simulink model "dbe_xaui_corr_32X"  (Simulink 7.1)
settings: Solver=ode45  StartTime=0.0  StopTime=1000  RelTol=1e-3
undefined symbols (not defined in the file or in its folder): iBOB
libraries: xbsIndex_r4 x455, xps_library x46, casper_library_misc x12, casper_library_sources x2, gavrt_library x1, simulink x1, casper_library_scopes x1
(part 1 of 4)
settings Model: Creator=rprimian  LastModifiedBy=Rurik A Primiani
settings DebuggingCC: SaveWithParameterizedLinksMsg=none  SignalResolutionControl=TryResolveAllWithWarning  MultiTaskDSMMsg=warning  MultiTaskCondExecSysMsg=none  StrictBusMsg=None
settings RTWCC: IncludeERTFirstTime=on
settings GRTTargetCC: TargetFcnLib=ansi_tfl_tmw.mat

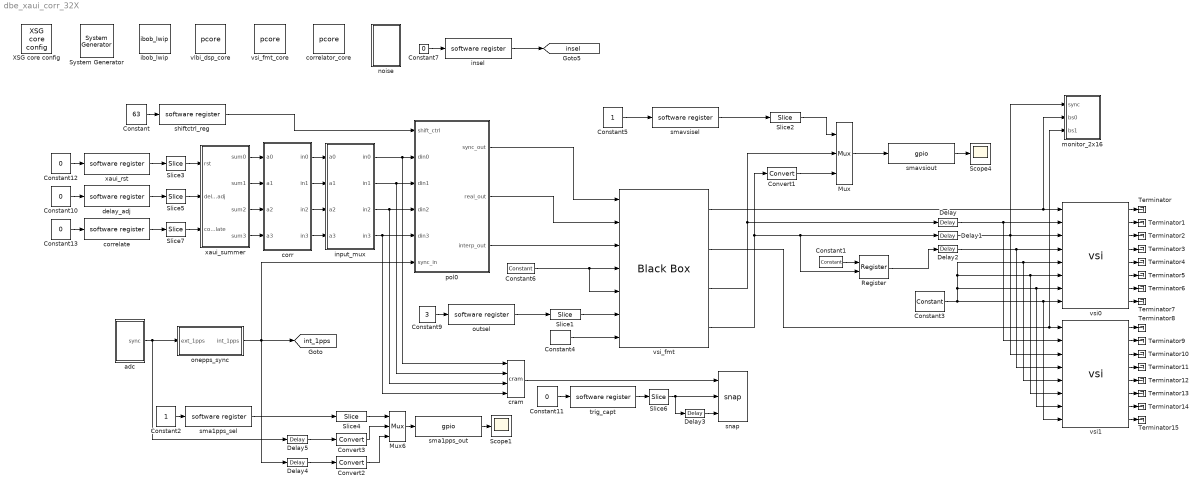
== system dbe_xaui_corr_32X ==
  " System Generator" : xbsIndex_r4/ System Generator  Tag=genX  SystemSampleTime=-1  xilinxfamily=virtex2p  part=xc2vp50  speed=-7  package=ff1152  synthesis_tool=XST  clock_wrapper=Clock Enables  directory=./dbe_xaui_corr_32X/sysgen  testbench=off  simulink_period=1  sysclk_period=3.9063  dcm_input_clock_period=10  incr_netlist=off  trim_vbits=Everywhere in SubSystem  dbl_ovrd=According to Block Masks  core_generation=According to Block Masks  run_coregen=off  deprecated_control=off  eval_field=0  block_type=sysgen
      settings: block_version=11.3
  Constant : Constant  Value=63  OutDataType=sfix(16)  OutScaling=2^0
  Constant1 : xbsIndex_r4/Constant  arith_type=Unsigned  const=1  n_bits=1  bin_pt=0  explicit_period=on  period=1  equ=P=C  opselect=C  inp2=PCIN>>17  opr=+  inp1=P  carry=CIN  dbl_ovrd=off  block_type=constant
      settings: block_version=11.3
  Constant{10..13} (4 alike) : Constant  Value=0  OutDataType=fixdt(1, 16)  OutScaling=2^0
  Constant2 : Constant  OutDataType=sfix(16)  OutScaling=2^0
  Constant3 : xbsIndex_r4/Constant  arith_type=Unsigned  const=0  n_bits=1  bin_pt=0  explicit_period=on  period=1  equ=P=C  opselect=C  inp2=PCIN>>17  opr=+  inp1=P  carry=CIN  dbl_ovrd=off  block_type=constant
      settings: block_version=11.3
  Constant4 : xbsIndex_r4/Constant  arith_type=Unsigned  const=6  n_bits=3  bin_pt=0  explicit_period=on  period=1  equ=P=C  opselect=C  inp2=PCIN>>17  opr=+  inp1=P  carry=CIN  dbl_ovrd=off  block_type=constant
      settings: block_version=11.3
  Constant5 : Constant  OutDataType=sfix(16)  OutScaling=2^0
  Constant6 : xbsIndex_r4/Constant  arith_type=Unsigned  const=0  n_bits=4  bin_pt=0  explicit_period=on  period=1  equ=P=C  opselect=C  inp2=PCIN>>17  opr=+  inp1=P  carry=CIN  dbl_ovrd=off  block_type=constant
      settings: block_version=11.3
  Constant7 : Constant  Value=0
  Constant9 : Constant  Value=3  OutDataType=sfix(16)  OutScaling=2^0
  Convert1 : xbsIndex_r4/Convert  arith_type=Unsigned  n_bits=1  bin_pt=0  quantization=Truncate  overflow=Wrap  latency=0  dbl_ovrd=off  pipeline=off  block_type=convert
      settings: xl_area=[0, 0, 0, 0, 0, 0, 0]  block_version=11.3
  Convert2 : xbsIndex_r4/Convert  arith_type=Unsigned  n_bits=1  bin_pt=0  quantization=Truncate  overflow=Wrap  latency=0  dbl_ovrd=off  pipeline=off  block_type=convert
      settings: xl_area=[0, 0, 0, 0, 0, 0, 0]  block_version=11.3
  Convert3 : xbsIndex_r4/Convert  arith_type=Unsigned  n_bits=1  bin_pt=0  quantization=Truncate  overflow=Wrap  latency=0  dbl_ovrd=off  pipeline=off  block_type=convert
      settings: xl_area=[0, 0, 0, 0, 0, 0, 0]  block_version=11.3
  Delay{,1,4..5} (4 alike) : xbsIndex_r4/Delay  en=off  latency=1  dbl_ovrd=off  reg_retiming=off  block_type=delay
      settings: xl_area=[0, 0, 0, 0, 0, 0, 0]  block_version=11.3
  Delay2 : xbsIndex_r4/Delay  en=off  latency=0  dbl_ovrd=off  reg_retiming=off  block_type=delay
      settings: xl_area=[0, 0, 0, 0, 0, 0, 0]  block_version=11.3
  Delay3 : xbsIndex_r4/Delay  en=off  latency=8  dbl_ovrd=off  reg_retiming=off  block_type=delay
      settings: xl_area=[0, 0, 0, 0, 0, 0, 0]  block_version=11.3
  Mux : xbsIndex_r4/Mux  inputs=2  en=off  latency=0  precision=Full  arith_type="Signed  (2's comp)"  n_bits=8  bin_pt=2  quantization=Truncate  overflow=Wrap  dbl_ovrd=off  block_type=mux
      settings: xl_area=[0, 0, 0, 0, 0, 0, 0]  block_version=11.3
  Mux6 : xbsIndex_r4/Mux  inputs=2  en=off  latency=0  precision=Full  arith_type="Signed  (2's comp)"  n_bits=8  bin_pt=2  quantization=Truncate  overflow=Wrap  dbl_ovrd=off  block_type=mux
      settings: xl_area=[0, 0, 0, 0, 0, 0, 0]  block_version=11.3
  Register : xbsIndex_r4/Register  init=0  rst=off  en=on  dbl_ovrd=off  block_type=register
      settings: xl_area=[0, 0, 0, 0, 0, 0, 0]  block_version=11.3
  Scope1 : Scope
      settings: TimeRange=94.87951807228916  YMin=0.5138408304498272  YMax=0.5276816608996542
  Scope4 : Scope
      settings: TimeRange=94.87951807228916  YMin=0.5138408304498272  YMax=0.5276816608996542  SaveName=ScopeData2
  Slice1 : xbsIndex_r4/Slice  nbits=2  boolean_output=off  mode=Lower Bit Location + Width  bit1=0  base1=MSB of Input  bit0=0  base0=LSB of Input  dbl_ovrd=off  block_type=slice
      settings: block_version=11.3
  Slice2 : xbsIndex_r4/Slice  nbits=1  boolean_output=off  mode=Lower Bit Location + Width  bit1=0  base1=MSB of Input  bit0=0  base0=LSB of Input  dbl_ovrd=off  block_type=slice
      settings: block_version=11.3
  Slice3 : xbsIndex_r4/Slice  nbits=1  boolean_output=on  mode=Lower Bit Location + Width  bit1=0  base1=MSB of Input  bit0=0  base0=LSB of Input  dbl_ovrd=off  block_type=slice
      settings: infoedit="Extracts a given range of bits from each input sample and presents it at the output.  The output type is ordinarily unsigned with binary point at zero, but can be Boolean when the slice is one bit wide.<P><P>Hardware notes: In hardware this block costs nothing."  block_version=10.1.3
  Slice4 : xbsIndex_r4/Slice  nbits=1  boolean_output=off  mode=Lower Bit Location + Width  bit1=0  base1=MSB of Input  bit0=0  base0=LSB of Input  dbl_ovrd=off  block_type=slice
      settings: block_version=11.3
  Slice5 : xbsIndex_r4/Slice  nbits=4  boolean_output=off  mode=Lower Bit Location + Width  bit1=0  base1=MSB of Input  bit0=0  base0=LSB of Input  dbl_ovrd=off  block_type=slice
      settings: infoedit="Extracts a given range of bits from each input sample and presents it at the output.  The output type is ordinarily unsigned with binary point at zero, but can be Boolean when the slice is one bit wide.<P><P>Hardware notes: In hardware this block costs nothing."  block_version=10.1.3
  Slice6 : xbsIndex_r4/Slice  nbits=4  boolean_output=on  mode=Lower Bit Location + Width  bit1=0  base1=MSB of Input  bit0=0  base0=LSB of Input  dbl_ovrd=off  block_type=slice
      settings: infoedit="Extracts a given range of bits from each input sample and presents it at the output.  The output type is ordinarily unsigned with binary point at zero, but can be Boolean when the slice is one bit wide.<P><P>Hardware notes: In hardware this block costs nothing."  block_version=10.1.3
  Slice7 : xbsIndex_r4/Slice  nbits=1  boolean_output=on  mode=Lower Bit Location + Width  bit1=0  base1=MSB of Input  bit0=0  base0=LSB of Input  dbl_ovrd=off  block_type=slice
      settings: infoedit="Extracts a given range of bits from each input sample and presents it at the output.  The output type is ordinarily unsigned with binary point at zero, but can be Boolean when the slice is one bit wide.<P><P>Hardware notes: In hardware this block costs nothing."  block_version=10.1.3
  Terminator{,1..15} (16 alike) : Terminator
  XSG core config : xps_library/XSG core config  Tag=xps:xsg  SystemSampleTime=-1  hw_sys=iBOB  ibob_linux=off  clk_src=adc0_clk  iBOB_clk_src=adc0_clk  BEE2_ctrl_clk_src=sys_clk  BEE2_usr_clk_src=sys_clk  ROACH_clk_src=adc0_clk  CORR_clk_src=sys_clk  gpio_clk_io_group=iBOB:gpio0  gpio_clk_bit_index=0  clk_rate=256  sample_period=1  synthesis_tool=XST  mpc_type=powerpc405
  adc : Subsystem
  corr : Subsystem
  correlate : xps_library/software register  Tag=xps:sw_reg  SystemSampleTime=-1  io_dir=From Processor  arith_type=Unsigned  bitwidth=32  bin_pt=0  sample_period=1  gw_name=dbe_xaui_corr_32X_correlate_user_data_out
      link override dbe_xaui_align_user_data_out: arith_type=Unsigned  n_bits=32  bin_pt=0  period=1
      link override dbe_xaui_corr_32X_correlate_user_data_out: arith_type=Unsigned  n_bits=32  bin_pt=0  period=1
      link override dbe_xaui_corr_correlate_user_data_out: arith_type=Unsigned  n_bits=32  bin_pt=0  period=1
      link override dbe_xaui_correlate_user_data_out: arith_type=Unsigned  n_bits=32  bin_pt=0  period=1
      link override dbe_xaui_realign_user_data_out: arith_type=Unsigned  n_bits=32  bin_pt=0  period=1
      link override xaui_rx_reset_user_data_out: arith_type=Unsigned  n_bits=32  bin_pt=0  period=1
  correlator_core : xps_library/pcore  Tag=xps:pcore  SystemSampleTime=-1  pcore_path=./correlator_core/correlator_core.ngc
  cram : gavrt_library/cram  SystemSampleTime=-1  num_slice=4
  delay_adj : xps_library/software register  Tag=xps:sw_reg  SystemSampleTime=-1  io_dir=From Processor  arith_type=Unsigned  bitwidth=32  bin_pt=0  sample_period=1  gw_name=dbe_xaui_corr_32X_delay_adj_user_data_out
      link override dbe_xaui_corr_32X_delay_adj_user_data_out: arith_type=Unsigned  n_bits=32  bin_pt=0  period=1
      link override dbe_xaui_corr_delay_adj_user_data_out: arith_type=Unsigned  n_bits=32  bin_pt=0  period=1
      link override dbe_xaui_delay_adj_user_data_out: arith_type=Unsigned  n_bits=32  bin_pt=0  period=1
      link override dbe_xaui_realign_user_data_out: arith_type=Unsigned  n_bits=32  bin_pt=0  period=1
      link override xaui_rx_reset_user_data_out: arith_type=Unsigned  n_bits=32  bin_pt=0  period=1
  ibob_lwip : xps_library/ibob_lwip  SystemSampleTime=-1
      link override macbits/convert: arith_type=Unsigned  n_bits=32  bin_pt=0
      link override machdr/dbe_xaui_corr_32X_ibob_lwip_machdr_gateway: arith_type=Unsigned  n_bits=20  bin_pt=0  period=sample_period
      link override machdr/dbe_xaui_corr_ibob_lwip_machdr_gateway: arith_type=Unsigned  n_bits=20  bin_pt=0  period=sample_period
  input_mux : Subsystem
  insel : xps_library/software register  Tag=xps:sw_reg  SystemSampleTime=-1  io_dir=From Processor  arith_type=Unsigned  bitwidth=32  bin_pt=0  sample_period=1  gw_name=dbe_xaui_corr_32X_insel_user_data_out
      link override dbe_adc_single_insel_user_data_out: arith_type=Unsigned  n_bits=32  bin_pt=0  period=1
      link override dbe_adc_single_shiftctrl_reg_user_data_out: arith_type=Unsigned  n_bits=32  bin_pt=0  period=1
      link override dbe_xaui_corr_32X_insel_user_data_out: arith_type=Unsigned  n_bits=32  bin_pt=0  period=1
      link override vlbipfb2_m3_ibob_shiftctrl_reg_user_data_out: arith_type=Unsigned  n_bits=32  bin_pt=0  period=1
      link override vlbipfb2_m3_roach_shiftctrl_reg_user_data_out: arith_type=Unsigned  n_bits=32  bin_pt=0  period=1
  monitor_2x16 : Subsystem  mask{sample_width=2}
      mask prompts: sample_width "Sample width"
  noise : Subsystem
  onepps_sync : Subsystem
  outsel : xps_library/software register  Tag=xps:sw_reg  SystemSampleTime=-1  io_dir=From Processor  arith_type=Unsigned  bitwidth=32  bin_pt=0  sample_period=1  gw_name=dbe_xaui_corr_32X_outsel_user_data_out
      link override dbe_adc_single_output_sel_user_data_out: arith_type=Unsigned  n_bits=32  bin_pt=0  period=1
      link override dbe_xaui_corr_32X_outsel_user_data_out: arith_type=Unsigned  n_bits=32  bin_pt=0  period=1
      link override vlbipfb2_m3_ibob_output_sel_user_data_out: arith_type=Unsigned  n_bits=32  bin_pt=0  period=1
      link override vlbipfb2_m3_roach_output_sel_user_data_out: arith_type=Unsigned  n_bits=32  bin_pt=0  period=1
  pol0 : Subsystem
  shiftctrl_reg : xps_library/software register  Tag=xps:sw_reg  SystemSampleTime=-1  io_dir=From Processor  arith_type=Unsigned  bitwidth=32  bin_pt=0  sample_period=1  gw_name=dbe_xaui_corr_32X_shiftctrl_reg_user_data_out
      link override dbe_xaui_corr_32X_shiftctrl_reg_user_data_out: arith_type=Unsigned  n_bits=32  bin_pt=0  period=1
      link override dbe_xaui_corr_shiftctrl_reg_user_data_out: arith_type=Unsigned  n_bits=32  bin_pt=0  period=1
      link override dbe_xaui_shiftctrl_reg_user_data_out: arith_type=Unsigned  n_bits=32  bin_pt=0  period=1
      link override vlbipfb2_m3_ibob_shiftctrl_reg_user_data_out: arith_type=Unsigned  n_bits=32  bin_pt=0  period=1
      link override vlbipfb2_m3_roach_shiftctrl_reg_user_data_out: arith_type=Unsigned  n_bits=32  bin_pt=0  period=1
  sma1pps_out : xps_library/gpio  Tag=xps:gpio  SystemSampleTime=-1  io_group=iBOB:sma  io_dir=out  arith_type=Unsigned  bitwidth=1  bin_pt=0  bit_index=0  sample_period=1  use_single_ended=off  use_ddr=off  reg_iob=on  reg_clk_phase=0  termination=None
      link override convert: arith_type=Unsigned  n_bits=1  bin_pt=0
  sma1pps_sel : xps_library/software register  Tag=xps:sw_reg  SystemSampleTime=-1  io_dir=From Processor  arith_type=Unsigned  bitwidth=32  bin_pt=0  sample_period=1  gw_name=dbe_xaui_corr_32X_sma1pps_sel_user_data_out
      link override dbe_xaui_corr_32X_sma1pps_sel_user_data_out: arith_type=Unsigned  n_bits=32  bin_pt=0  period=1
      link override dbe_xaui_corr_sma1pps_sel_user_data_out: arith_type=Unsigned  n_bits=32  bin_pt=0  period=1
      link override dbe_xaui_corr_smasel_user_data_out: arith_type=Unsigned  n_bits=32  bin_pt=0  period=1
      link override dbe_xaui_smasel_user_data_out: arith_type=Unsigned  n_bits=32  bin_pt=0  period=1
      link override vlbipfb2_m3_ibob_smasel_user_data_out: arith_type=Unsigned  n_bits=32  bin_pt=0  period=1
      link override vlbipfb2_m3_roach_smasel_user_data_out: arith_type=Unsigned  n_bits=32  bin_pt=0  period=1
  smavsiout : xps_library/gpio  Tag=xps:gpio  SystemSampleTime=-1  io_group=iBOB:sma  io_dir=out  arith_type=Unsigned  bitwidth=1  bin_pt=0  bit_index=1  sample_period=1  use_single_ended=off  use_ddr=off  reg_iob=on  reg_clk_phase=0  termination=None
      link override convert: arith_type=Unsigned  n_bits=1  bin_pt=0
  smavsisel : xps_library/software register  Tag=xps:sw_reg  SystemSampleTime=-1  io_dir=From Processor  arith_type=Unsigned  bitwidth=32  bin_pt=0  sample_period=1  gw_name=dbe_xaui_corr_32X_smavsisel_user_data_out
      link override dbe_adc_single_smasel_user_data_out: arith_type=Unsigned  n_bits=32  bin_pt=0  period=1
      link override dbe_xaui_corr_32X_smavsisel_user_data_out: arith_type=Unsigned  n_bits=32  bin_pt=0  period=1
      link override vlbipfb2_m3_ibob_smasel_user_data_out: arith_type=Unsigned  n_bits=32  bin_pt=0  period=1
      link override vlbipfb2_m3_roach_smasel_user_data_out: arith_type=Unsigned  n_bits=32  bin_pt=0  period=1
  snap : casper_library_scopes/snap  SystemSampleTime=-1  nsamples=11
      link override addr/convert: arith_type=Unsigned  n_bits=32  bin_pt=0
      link override bram/convert_din: arith_type=Unsigned
      link override bram/dbe_xaui_corr_32X_snap_bram_data_out: arith_type=Unsigned
      link override bram/dbe_xaui_corr_snap_bram_data_out: arith_type=Unsigned
      link override bram/dbe_xaui_snap_bram_data_out: arith_type=Unsigned
      link override bram/mem/sim_data_in: arith_type=Unsigned
      link override ctrl/dbe_xaui_corr_32X_snap_ctrl_user_data_out: arith_type=Unsigned  n_bits=32  bin_pt=0  period=1
      link override ctrl/dbe_xaui_corr_snap_ctrl_user_data_out: arith_type=Unsigned  n_bits=32  bin_pt=0  period=1
      link override ctrl/dbe_xaui_snap_ctrl_user_data_out: arith_type=Unsigned  n_bits=32  bin_pt=0  period=1
  trig_capt : xps_library/software register  Tag=xps:sw_reg  SystemSampleTime=-1  io_dir=From Processor  arith_type=Unsigned  bitwidth=32  bin_pt=0  sample_period=1  gw_name=dbe_xaui_corr_32X_trig_capt_user_data_out
      link override dbe_xaui_corr_32X_trig_capt_user_data_out: arith_type=Unsigned  n_bits=32  bin_pt=0  period=1
      link override dbe_xaui_corr_trig_capt_user_data_out: arith_type=Unsigned  n_bits=32  bin_pt=0  period=1
      link override dbe_xaui_delay_adj_user_data_out: arith_type=Unsigned  n_bits=32  bin_pt=0  period=1
      link override dbe_xaui_realign_user_data_out: arith_type=Unsigned  n_bits=32  bin_pt=0  period=1
      link override dbe_xaui_trig_capt_user_data_out: arith_type=Unsigned  n_bits=32  bin_pt=0  period=1
      link override xaui_rx_reset_user_data_out: arith_type=Unsigned  n_bits=32  bin_pt=0  period=1
  vlbi_dsp_core : xps_library/pcore  Tag=xps:pcore  SystemSampleTime=-1  pcore_path=vlbi_dsp_core/vlbi_dsp_core.ngc
  vsi0 : xps_library/vsi  Tag=xps:vsi  SystemSampleTime=-1  connector=MDR  arith_type=Unsigned  bin_pt=0  sample_period=1
      link override convert_bs: arith_type=Unsigned  n_bits=32  bin_pt=0
  vsi1 : xps_library/vsi  Tag=xps:vsi  SystemSampleTime=-1  connector=ZDOK 1  arith_type=Unsigned  bin_pt=0  sample_period=1
      link override convert_bs: arith_type=Unsigned  n_bits=32  bin_pt=0
  vsi_fmt : xbsIndex_r4/Black Box  init_code=vsi_fmt_core_config  sim_method=Inactive  block_type=blackbox2
      settings: infoedit="Incorporates black box HDL and simulation model into a System Generator design.<P><P>You must supply a Black Box with certain information about the HDL component you would like to bring into System Generator. This information is provided through a Matlab function.<P><P>When \"Simulation mode\" is set to \"Inactive\", you will typically want to provide a separate simulation model by using a Simulation Multiplexer.<P>When \"Simulation mode\" is set to \"External co-simulator\", you must include a ModelSim block in the design."  block_version=10.1.3
  vsi_fmt_core : xps_library/pcore  Tag=xps:pcore  SystemSampleTime=-1  pcore_path=vsi_fmt_core/vsi_fmt_core.ngc
  xaui_rst : xps_library/software register  Tag=xps:sw_reg  SystemSampleTime=-1  io_dir=From Processor  arith_type=Unsigned  bitwidth=32  bin_pt=0  sample_period=1  gw_name=dbe_xaui_corr_32X_xaui_rst_user_data_out
      link override dbe_xaui_corr_32X_xaui_rst_user_data_out: arith_type=Unsigned  n_bits=32  bin_pt=0  period=1
      link override dbe_xaui_corr_xaui_rst_user_data_out: arith_type=Unsigned  n_bits=32  bin_pt=0  period=1
      link override dbe_xaui_xaui_rst_user_data_out: arith_type=Unsigned  n_bits=32  bin_pt=0  period=1
      link override xaui_rx_reset_user_data_out: arith_type=Unsigned  n_bits=32  bin_pt=0  period=1
  xaui_summer : Subsystem
  tag scope: insel=global, int_1pps=global
  wires:
  Constant/1 -> shiftctrl_reg/1
  adc/1(sync) -> onepps_sync/1(ext_1pps), Delay5/1
  shiftctrl_reg/1 -> pol0/1(shift_ctrl)
  onepps_sync/1(int_1pps) -> pol0/6(sync_in), [int_1pps], Delay4/1
  Constant12/1 -> xaui_rst/1
  xaui_rst/1 -> Slice3/1
  Slice3/1 -> xaui_summer/1(rst)
  Constant10/1 -> delay_adj/1
  delay_adj/1 -> Slice5/1
  Slice5/1 -> xaui_summer/2(delay_adj)
  Constant13/1 -> correlate/1
  correlate/1 -> Slice7/1
  Slice7/1 -> xaui_summer/3(correlate)
  Mux6/1 -> sma1pps_out/1
  sma1pps_sel/1 -> Slice4/1
  Constant2/1 -> sma1pps_sel/1
  Convert2/1 -> Mux6/3
  Slice4/1 -> Mux6/1
  sma1pps_out/1 -> Scope1/1
  Convert3/1 -> Mux6/2
  vsi_fmt/4 -> Delay1/1, Register/2, Convert1/1
  Constant3/1 -> vsi0/6, vsi1/6, vsi0/5, vsi1/5, vsi0/7, vsi1/7, vsi0/8, vsi1/8
  Constant1/1 -> Register/1
  Register/1 -> Delay2/1
  Mux/1 -> smavsiout/1
  smavsisel/1 -> Slice2/1
  Constant5/1 -> smavsisel/1
  Convert1/1 -> Mux/3
  Slice2/1 -> Mux/1
  smavsiout/1 -> Scope4/1
  Constant9/1 -> outsel/1
  Delay/1 -> vsi0/2, vsi1/2
  Delay1/1 -> monitor_2x16/1(sync), vsi0/3, vsi1/3
  Delay2/1 -> vsi0/4, vsi1/4
  input_mux/1(in0) -> pol0/2(din0), cram/1
  input_mux/2(in1) -> pol0/3(din1), cram/2
  input_mux/3(in2) -> pol0/4(din2), cram/3
  input_mux/4(in3) -> pol0/5(din3), cram/4
  vsi_fmt/3 -> Mux/2, Delay/1
  vsi_fmt/1 -> vsi0/1, monitor_2x16/2(bs0)
  vsi_fmt/2 -> monitor_2x16/3(bs1), vsi1/1
  pol0/1(sync_out) -> vsi_fmt/1
  pol0/2(real_out) -> vsi_fmt/2
  pol0/3(interp_out) -> vsi_fmt/3
  Constant6/1 -> vsi_fmt/4, vsi_fmt/5
  outsel/1 -> Slice1/1
  Constant4/1 -> vsi_fmt/7
  Slice1/1 -> vsi_fmt/6
  cram/1 -> snap/1
  Constant11/1 -> trig_capt/1
  trig_capt/1 -> Slice6/1
  Delay3/1 -> snap/3
  Slice6/1 -> snap/2, Delay3/1
  Constant7/1 -> insel/1
  insel/1 -> [insel]
  vsi0/1 -> Terminator/1
  vsi0/2 -> Terminator1/1
  vsi0/3 -> Terminator2/1
  vsi0/4 -> Terminator3/1
  vsi0/5 -> Terminator4/1
  vsi0/6 -> Terminator5/1
  vsi0/7 -> Terminator6/1
  vsi0/8 -> Terminator7/1
  vsi1/1 -> Terminator8/1
  vsi1/2 -> Terminator9/1
  vsi1/3 -> Terminator10/1
  vsi1/4 -> Terminator11/1
  vsi1/5 -> Terminator12/1
  vsi1/6 -> Terminator13/1
  vsi1/7 -> Terminator14/1
  vsi1/8 -> Terminator15/1
  Delay5/1 -> Convert3/1
  Delay4/1 -> Convert2/1
  xaui_summer/1(sum0) -> corr/1(a0)
  xaui_summer/2(sum1) -> corr/2(a1)
  xaui_summer/3(sum2) -> corr/3(a2)
  xaui_summer/4(sum3) -> corr/4(a3)
  corr/1(in0) -> input_mux/1(a0)
  corr/2(in1) -> input_mux/2(a1)
  corr/3(in2) -> input_mux/3(a2)
  corr/4(in3) -> input_mux/4(a3)

== system dbe_xaui_corr_32X/adc ==
  Constant10 : Constant  OutDataType=sfix(16)  OutScaling=2^0  SampleTime=0.25
  Pulse Generator : DiscretePulseGenerator  Period=2560  PhaseDelay=20  SampleTime=0.25
  Sine Wave : Sin  Amplitude=.8  Frequency=2*pi*119/256  Samples=2*pi*129/1024  SampleTime=1/4
  Sine Wave1 : Sin  Amplitude=.8  Frequency=2*pi*77/256  Samples=2*pi*129/1024  SampleTime=1/4
  Terminator{,1..6,8..12} (12 alike) : Terminator
  adc : xps_library/adc  Tag=xps:adc  SystemSampleTime=-1  adc_brd=adc0  adc_clk_rate=1024  adc_interleave=off  sample_period=1
  sync : Outport
  tag scope: adc0=global, adc1=global, adc2=global, adc3=global
  wires:
  Constant10/1 -> adc/4
  Pulse Generator/1 -> adc/3
  Sine Wave/1 -> adc/1
  adc/9 -> Terminator/1
  adc/10 -> Terminator1/1
  adc/11 -> Terminator3/1
  adc/12 -> Terminator8/1
  adc/14 -> Terminator9/1
  adc/15 -> Terminator10/1
  adc/16 -> Terminator11/1
  adc/17 -> Terminator12/1
  Sine Wave1/1 -> adc/2
  adc/5 -> Terminator2/1
  adc/6 -> Terminator4/1
  adc/7 -> Terminator5/1
  adc/8 -> Terminator6/1
  adc/1 -> [adc0]
  adc/2 -> [adc1]
  adc/3 -> [adc2]
  adc/4 -> [adc3]
  adc/13 -> sync/1

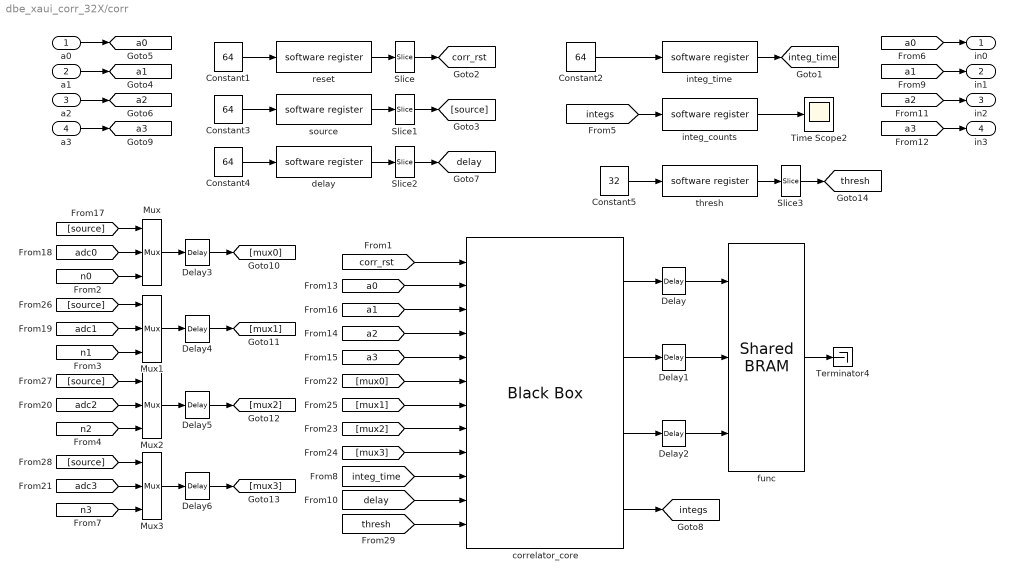
== system dbe_xaui_corr_32X/corr ==
  a0 : Inport
  a1 : Inport  Port=2
  a2 : Inport  Port=3
  a3 : Inport  Port=4
  Constant{1..4} (4 alike) : Constant  Value=64  OutDataType=fixdt(1, 16)  OutScaling=2^0
  Constant5 : Constant  Value=32  OutDataType=fixdt(1, 16)  OutScaling=2^0
  Delay{,1..6} (7 alike) : xbsIndex_r4/Delay  en=off  latency=1  dbl_ovrd=off  reg_retiming=off  block_type=delay
  Mux{,1..3} (4 alike) : xbsIndex_r4/Mux  inputs=2  en=off  latency=1  precision=Full  arith_type=Unsigned  n_bits=16  bin_pt=14  quantization=Truncate  overflow=Wrap  dbl_ovrd=off  block_type=mux
  Slice : xbsIndex_r4/Slice  nbits=1  boolean_output=on  mode=Lower Bit Location + Width  bit1=0  base1=MSB of Input  bit0=0  base0=LSB of Input  dbl_ovrd=off  block_type=slice
      settings: infoedit="Extracts a given range of bits from each input sample and presents it at the output.  The output type is ordinarily unsigned with binary point at zero, but can be Boolean when the slice is one bit wide.<P><P>Hardware notes: In hardware this block costs nothing."  block_version=10.1.3
  Slice1 : xbsIndex_r4/Slice  nbits=1  boolean_output=on  mode=Lower Bit Location + Width  bit1=0  base1=MSB of Input  bit0=0  base0=LSB of Input  dbl_ovrd=off  block_type=slice
      settings: infoedit="Extracts a given range of bits from each input sample and presents it at the output.  The output type is ordinarily unsigned with binary point at zero, but can be Boolean when the slice is one bit wide.<P><P>Hardware notes: In hardware this block costs nothing."  block_version=10.1.3
  Slice2 : xbsIndex_r4/Slice  nbits=11  boolean_output=off  mode=Lower Bit Location + Width  bit1=0  base1=MSB of Input  bit0=0  base0=LSB of Input  dbl_ovrd=off  block_type=slice
      settings: infoedit="Extracts a given range of bits from each input sample and presents it at the output.  The output type is ordinarily unsigned with binary point at zero, but can be Boolean when the slice is one bit wide.<P><P>Hardware notes: In hardware this block costs nothing."  block_version=10.1.3
  Slice3 : xbsIndex_r4/Slice  nbits=7  boolean_output=off  mode=Lower Bit Location + Width  bit1=0  base1=MSB of Input  bit0=0  base0=LSB of Input  dbl_ovrd=off  block_type=slice
      settings: infoedit="Extracts a given range of bits from each input sample and presents it at the output.  The output type is ordinarily unsigned with binary point at zero, but can be Boolean when the slice is one bit wide.<P><P>Hardware notes: In hardware this block costs nothing."  block_version=10.1.3
  Terminator4 : Terminator
  Time Scope2 : Scope
      settings: YMin=0  YMax=32.5  SaveName=ScopeData3  DataFormat=Structure
  correlator_core : xbsIndex_r4/Black Box  init_code=correlator_core_config  sim_method=Inactive  block_type=blackbox2
      settings: infoedit="Incorporates black box HDL and simulation model into a System Generator design.<P><P>You must supply a Black Box with certain information about the HDL component you would like to bring into System Generator. This information is provided through a Matlab function.<P><P>When \"Simulation mode\" is set to \"Inactive\", you will typically want to provide a separate simulation model by using a Simulation Multiplexer.<P>When \"Simulation mode\" is set to \"External co-simulator\", you must include a ModelSim block in the design."  block_version=10.1.3
  delay : xps_library/software register  Tag=xps:sw_reg  SystemSampleTime=-1  io_dir=From Processor  arith_type=Unsigned  bitwidth=32  bin_pt=0  sample_period=1  gw_name=dbe_xaui_corr_32X_corr_delay_user_data_out
      link override correlator_2bit_bee2_integ_time_user_data_out: arith_type=Unsigned  n_bits=32  bin_pt=0  period=1
      link override correlator_2bit_bee2_x2_integ_time_user_data_out: arith_type=Unsigned  n_bits=32  bin_pt=0  period=1
      link override correlator_2bit_ibob_integ_time_user_data_out: arith_type=Unsigned  n_bits=32  bin_pt=0  period=1
      link override dbe_xaui_corr_32X_corr_delay_user_data_out: arith_type=Unsigned  n_bits=32  bin_pt=0  period=1
      link override dbe_xaui_corr_corr_delay_user_data_out: arith_type=Unsigned  n_bits=32  bin_pt=0  period=1
      link override dbe_xaui_corr_corr_integ_time_user_data_out: arith_type=Unsigned  n_bits=32  bin_pt=0  period=1
      link override dbe_xaui_corr_corr_integ_user_data_out: arith_type=Unsigned  n_bits=32  bin_pt=0  period=1
      link override dbe_xaui_corr_new_corr_integ_user_data_out: arith_type=Unsigned  n_bits=32  bin_pt=0  period=1
  func : xps_library/Shared BRAM  Tag=xps:bram  SystemSampleTime=-1  arith_type="Signed  (2's comp)"  addr_width=11  data_width=32  data_bin_pt=0  init_vals=0  sample_rate=1
      link override convert_din: arith_type="Signed  (2's comp)"
      link override correlator_2bit_bee2_output_corr0_data_out: arith_type=Unsigned
      link override correlator_2bit_bee2_x2_output_corr01_data_out: arith_type=Unsigned
      link override correlator_2bit_bee2_x2_output_corr0_data_out: arith_type=Unsigned
      link override correlator_2bit_ibob_output_corr0_data_out: arith_type=Unsigned
      link override cross_correlator_test_corr_out_data_out: arith_type="Signed  (2's comp)"
      link override cross_correlator_test_input_data1_data_out: arith_type=Unsigned
      link override dbe_xaui_corr_32X_corr_func_data_out: arith_type="Signed  (2's comp)"
      link override dbe_xaui_corr_corr_func_data_out: arith_type="Signed  (2's comp)"
      link override dbe_xaui_corr_new_xaui_summer_summer_output_corr_data_out: arith_type="Signed  (2's comp)"
      link override dbe_xaui_corr_xaui_summer_summer_output_corr_data_out: arith_type="Signed  (2's comp)"
      link override mem/sim_data_in: arith_type="Signed  (2's comp)"
  integ_counts : xps_library/software register  Tag=xps:sw_reg  SystemSampleTime=-1  io_dir=To Processor  arith_type=Unsigned  bitwidth=32  bin_pt=0  sample_period=1  gw_name=dbe_xaui_corr_32X_corr_integ_counts_user_data_in
      link override convert: arith_type=Unsigned  n_bits=32  bin_pt=0
  integ_time : xps_library/software register  Tag=xps:sw_reg  SystemSampleTime=-1  io_dir=From Processor  arith_type=Unsigned  bitwidth=32  bin_pt=0  sample_period=1  gw_name=dbe_xaui_corr_32X_corr_integ_time_user_data_out
      link override correlator_2bit_bee2_integ_time_user_data_out: arith_type=Unsigned  n_bits=32  bin_pt=0  period=1
      link override correlator_2bit_bee2_x2_integ_time_user_data_out: arith_type=Unsigned  n_bits=32  bin_pt=0  period=1
      link override correlator_2bit_ibob_integ_time_user_data_out: arith_type=Unsigned  n_bits=32  bin_pt=0  period=1
      link override dbe_xaui_corr_32X_corr_integ_time_user_data_out: arith_type=Unsigned  n_bits=32  bin_pt=0  period=1
      link override dbe_xaui_corr_corr_integ_time_user_data_out: arith_type=Unsigned  n_bits=32  bin_pt=0  period=1
      link override dbe_xaui_corr_corr_integ_user_data_out: arith_type=Unsigned  n_bits=32  bin_pt=0  period=1
      link override dbe_xaui_corr_new_corr_integ_user_data_out: arith_type=Unsigned  n_bits=32  bin_pt=0  period=1
  reset : xps_library/software register  Tag=xps:sw_reg  SystemSampleTime=-1  io_dir=From Processor  arith_type=Unsigned  bitwidth=32  bin_pt=0  sample_period=1  gw_name=dbe_xaui_corr_32X_corr_reset_user_data_out
      link override correlator_2bit_bee2_integ_time_user_data_out: arith_type=Unsigned  n_bits=32  bin_pt=0  period=1
      link override correlator_2bit_bee2_x2_integ_time_user_data_out: arith_type=Unsigned  n_bits=32  bin_pt=0  period=1
      link override correlator_2bit_ibob_integ_time_user_data_out: arith_type=Unsigned  n_bits=32  bin_pt=0  period=1
      link override dbe_xaui_corr_32X_corr_reset_user_data_out: arith_type=Unsigned  n_bits=32  bin_pt=0  period=1
      link override dbe_xaui_corr_corr_integ_user_data_out: arith_type=Unsigned  n_bits=32  bin_pt=0  period=1
      link override dbe_xaui_corr_corr_reset_user_data_out: arith_type=Unsigned  n_bits=32  bin_pt=0  period=1
      link override dbe_xaui_corr_new_corr_integ_user_data_out: arith_type=Unsigned  n_bits=32  bin_pt=0  period=1
  source : xps_library/software register  Tag=xps:sw_reg  SystemSampleTime=-1  io_dir=From Processor  arith_type=Unsigned  bitwidth=32  bin_pt=0  sample_period=1  gw_name=dbe_xaui_corr_32X_corr_source_user_data_out
      link override correlator_2bit_bee2_integ_time_user_data_out: arith_type=Unsigned  n_bits=32  bin_pt=0  period=1
      link override correlator_2bit_bee2_x2_integ_time_user_data_out: arith_type=Unsigned  n_bits=32  bin_pt=0  period=1
      link override correlator_2bit_ibob_integ_time_user_data_out: arith_type=Unsigned  n_bits=32  bin_pt=0  period=1
      link override dbe_xaui_corr_32X_corr_source_user_data_out: arith_type=Unsigned  n_bits=32  bin_pt=0  period=1
      link override dbe_xaui_corr_corr_integ_time_user_data_out: arith_type=Unsigned  n_bits=32  bin_pt=0  period=1
      link override dbe_xaui_corr_corr_integ_user_data_out: arith_type=Unsigned  n_bits=32  bin_pt=0  period=1
      link override dbe_xaui_corr_corr_source_user_data_out: arith_type=Unsigned  n_bits=32  bin_pt=0  period=1
      link override dbe_xaui_corr_new_corr_integ_user_data_out: arith_type=Unsigned  n_bits=32  bin_pt=0  period=1
  thresh : xps_library/software register  Tag=xps:sw_reg  SystemSampleTime=-1  io_dir=From Processor  arith_type=Unsigned  bitwidth=32  bin_pt=0  sample_period=1  gw_name=dbe_xaui_corr_32X_corr_thresh_user_data_out
      link override correlator_2bit_bee2_integ_time_user_data_out: arith_type=Unsigned  n_bits=32  bin_pt=0  period=1
      link override correlator_2bit_bee2_x2_integ_time_user_data_out: arith_type=Unsigned  n_bits=32  bin_pt=0  period=1
      link override correlator_2bit_ibob_integ_time_user_data_out: arith_type=Unsigned  n_bits=32  bin_pt=0  period=1
      link override dbe_xaui_corr_32X_corr_thresh_user_data_out: arith_type=Unsigned  n_bits=32  bin_pt=0  period=1
      link override dbe_xaui_corr_corr_delay_user_data_out: arith_type=Unsigned  n_bits=32  bin_pt=0  period=1
      link override dbe_xaui_corr_corr_integ_time_user_data_out: arith_type=Unsigned  n_bits=32  bin_pt=0  period=1
      link override dbe_xaui_corr_corr_integ_user_data_out: arith_type=Unsigned  n_bits=32  bin_pt=0  period=1
      link override dbe_xaui_corr_corr_thresh_user_data_out: arith_type=Unsigned  n_bits=32  bin_pt=0  period=1
      link override dbe_xaui_corr_new_corr_integ_user_data_out: arith_type=Unsigned  n_bits=32  bin_pt=0  period=1
  in0 : Outport
  in1 : Outport  Port=2
  in2 : Outport  Port=3
  in3 : Outport  Port=4
  tag scope: a0=global, a1=global, a2=global, a3=global, corr_rst=global, delay=global, integ_time=global, integs=global, thresh=global
  wires:
  Constant2/1 -> integ_time/1
  integ_counts/1 -> Time Scope2/1
  integ_time/1 -> [integ_time]
  [integs] -> integ_counts/1
  func/1 -> Terminator4/1
  Constant1/1 -> reset/1
  reset/1 -> Slice/1
  Slice/1 -> [corr_rst]
  Constant3/1 -> source/1
  source/1 -> Slice1/1
  [corr_rst] -> correlator_core/1
  a0/1 -> [a0]
  a1/1 -> [a1]
  a2/1 -> [a2]
  a3/1 -> [a3]
  [a0] -> in0/1
  [a1] -> in1/1
  [a2] -> in2/1
  [a3] -> in3/1
  [a0] -> correlator_core/2
  [a1] -> correlator_core/3
  [a2] -> correlator_core/4
  [a3] -> correlator_core/5
  [n0] -> Mux/3
  [n1] -> Mux1/3
  [n2] -> Mux2/3
  [n3] -> Mux3/3
  [adc0] -> Mux/2
  [adc1] -> Mux1/2
  [adc2] -> Mux2/2
  [adc3] -> Mux3/2
  Mux/1 -> Delay3/1
  Mux1/1 -> Delay4/1
  Mux2/1 -> Delay5/1
  Mux3/1 -> Delay6/1
  [mux0] -> correlator_core/6
  [mux1] -> correlator_core/7
  [mux2] -> correlator_core/8
  [mux3] -> correlator_core/9
  [source] -> Mux/1
  [source] -> Mux1/1
  [source] -> Mux2/1
  Slice1/1 -> [source]
  [source] -> Mux3/1
  Constant4/1 -> delay/1
  delay/1 -> Slice2/1
  Slice2/1 -> [delay]
  correlator_core/1 -> Delay/1
  correlator_core/2 -> Delay1/1
  correlator_core/3 -> Delay2/1
  [integ_time] -> correlator_core/10
  [delay] -> correlator_core/11
  correlator_core/4 -> [integs]
  Delay/1 -> func/1
  Delay1/1 -> func/2
  Delay2/1 -> func/3
  [thresh] -> correlator_core/12
  Constant5/1 -> thresh/1
  thresh/1 -> Slice3/1
  Slice3/1 -> [thresh]
  Delay3/1 -> [mux0]
  Delay4/1 -> [mux1]
  Delay5/1 -> [mux2]
  Delay6/1 -> [mux3]

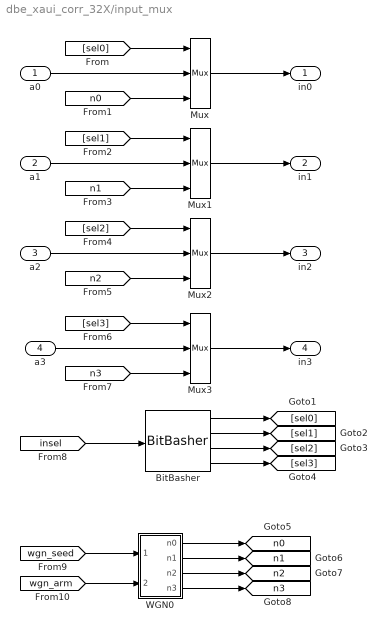
== system dbe_xaui_corr_32X/input_mux ==
  a0 : Inport
  a1 : Inport  Port=2
  a2 : Inport  Port=3
  a3 : Inport  Port=4
  BitBasher : xbsIndex_r4/BitBasher  bitexpr=|  display_expr=off  sr_1=1  arith_type1=Unsigned  bin_pt1=0  sr_2=2  arith_type2=Unsigned  bin_pt2=0  sr_3=3  arith_type3=Unsigned  bin_pt3=0  sr_4=4  arith_type4=Unsigned  bin_pt4=0  dbl_ovrd=off  block_type=bitbasher
      | <html><head><meta name="qrichtext" content="1" /><style type="text/css">
      | p, li { white-space: pre-wrap; }
      | </style></head><body style=" font-family:'MS Shell Dlg 2'; font-size:8.25pt; font-weight:400; font-style:normal;">
      | <p style=" margin-top:12px; margin-bottom:12px; margin-left:0px; margin-right:0px; -qt-block-indent:0; text-indent:0px; font-family:'MS Shell Dlg'; font-size:8pt;">sel0={insel[0]}<br />sel1={insel[1]}<br />sel2={insel[2]}<br />sel3={insel[3]}<br /></p></body></html>
      settings: block_version=10.1.3
  Mux{,1..3} (4 alike) : xbsIndex_r4/Mux  inputs=2  en=off  latency=0  precision=Full  arith_type=Unsigned  n_bits=16  bin_pt=14  quantization=Truncate  overflow=Wrap  dbl_ovrd=off  block_type=mux
  WGN0 : Subsystem
  in0 : Outport
  in1 : Outport  Port=2
  in2 : Outport  Port=3
  in3 : Outport  Port=4
  tag scope: n0=global, n1=global, n2=global, n3=global
  wires:
  Mux/1 -> in0/1
  BitBasher/1 -> [sel0]
  BitBasher/2 -> [sel1]
  BitBasher/3 -> [sel2]
  BitBasher/4 -> [sel3]
  [sel0] -> Mux/1
  WGN0/1(n0) -> [n0]
  WGN0/2(n1) -> [n1]
  WGN0/3(n2) -> [n2]
  WGN0/4(n3) -> [n3]
  a0/1 -> Mux/2
  [n0] -> Mux/3
  Mux1/1 -> in1/1
  [sel1] -> Mux1/1
  a1/1 -> Mux1/2
  [n1] -> Mux1/3
  Mux2/1 -> in2/1
  [sel2] -> Mux2/1
  a2/1 -> Mux2/2
  [n2] -> Mux2/3
  Mux3/1 -> in3/1
  [sel3] -> Mux3/1
  a3/1 -> Mux3/2
  [n3] -> Mux3/3
  [insel] -> BitBasher/1
  [wgn_seed] -> WGN0/1(seed)
  [wgn_arm] -> WGN0/2(arm)

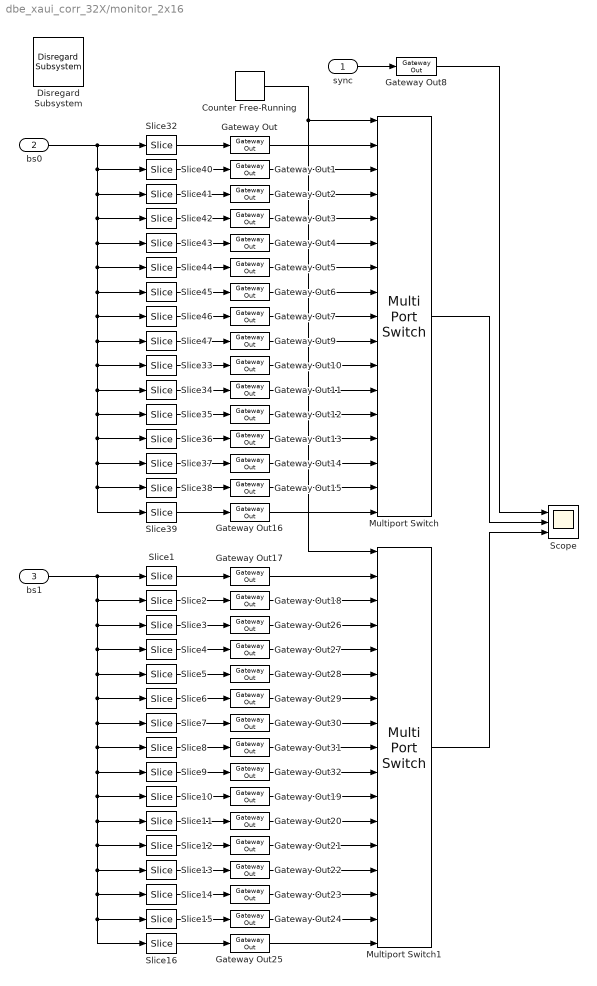
== system dbe_xaui_corr_32X/monitor_2x16 ==
  sync : Inport  OutDataType=sfix(16)  OutScaling=2^0
  bs0 : Inport  Port=2  OutDataType=sfix(16)  OutScaling=2^0
  bs1 : Inport  Port=3  OutDataType=sfix(16)  OutScaling=2^0
  Counter Free-Running : simulink/Sources/Counter Free-Running  SystemSampleTime=-1  NumBits=4  tsamp=1/16
  Disregard Subsystem : xbsIndex_r4/Disregard Subsystem  Tag=discardX  block_type=disregard
      settings: block_version=11.3
  Gateway Out{,1..32} (33 alike) : xbsIndex_r4/Gateway Out  hdl_port=off  timing_constraint=None  locs_specified=off  LOCs={}  block_type=gatewayout
      settings: infoedit="Gateway out block.  Converts Xilinx fixed point inputs into ouputs of type Simulink integer, double, or fixed point.<br><br>Hardware notes:  In hardware these blocks become top level output ports or are discarded, depending on how they are configured."  xl_area=[0, 0, 0, 0, 0, 0, 0]  block_version=11.3
  Multiport Switch : MultiPortSwitch  Inputs=16  zeroidx=on  SampleTime=1/16
  Multiport Switch1 : MultiPortSwitch  Inputs=16  zeroidx=on  SampleTime=1/16
  Scope : Scope  NumInputPorts=3
      settings: YMin=-5~-5~-5  YMax=5~5~5
  Slice1 : xbsIndex_r4/Slice  nbits=sample_width  boolean_output=off  mode=Upper Bit Location + Width  bit1=sample_width * 0  base1=MSB of Input  bit0=0  base0=LSB of Input  dbl_ovrd=off  block_type=slice
      settings: block_version=11.3
  Slice10 : xbsIndex_r4/Slice  nbits=sample_width  boolean_output=off  mode=Upper Bit Location + Width  bit1=sample_width * -9  base1=MSB of Input  bit0=0  base0=LSB of Input  dbl_ovrd=off  block_type=slice
      settings: block_version=11.3
  Slice11 : xbsIndex_r4/Slice  nbits=sample_width  boolean_output=off  mode=Upper Bit Location + Width  bit1=sample_width * -10  base1=MSB of Input  bit0=0  base0=LSB of Input  dbl_ovrd=off  block_type=slice
      settings: block_version=11.3
  Slice12 : xbsIndex_r4/Slice  nbits=sample_width  boolean_output=off  mode=Upper Bit Location + Width  bit1=sample_width * -11  base1=MSB of Input  bit0=0  base0=LSB of Input  dbl_ovrd=off  block_type=slice
      settings: block_version=11.3
  Slice13 : xbsIndex_r4/Slice  nbits=sample_width  boolean_output=off  mode=Upper Bit Location + Width  bit1=sample_width * -12  base1=MSB of Input  bit0=0  base0=LSB of Input  dbl_ovrd=off  block_type=slice
      settings: block_version=11.3
  Slice14 : xbsIndex_r4/Slice  nbits=sample_width  boolean_output=off  mode=Upper Bit Location + Width  bit1=sample_width * -13  base1=MSB of Input  bit0=0  base0=LSB of Input  dbl_ovrd=off  block_type=slice
      settings: block_version=11.3
  Slice15 : xbsIndex_r4/Slice  nbits=sample_width  boolean_output=off  mode=Upper Bit Location + Width  bit1=sample_width * -14  base1=MSB of Input  bit0=0  base0=LSB of Input  dbl_ovrd=off  block_type=slice
      settings: block_version=11.3
  Slice16 : xbsIndex_r4/Slice  nbits=sample_width  boolean_output=off  mode=Upper Bit Location + Width  bit1=sample_width * -15  base1=MSB of Input  bit0=0  base0=LSB of Input  dbl_ovrd=off  block_type=slice
      settings: block_version=11.3
  Slice2 : xbsIndex_r4/Slice  nbits=sample_width  boolean_output=off  mode=Upper Bit Location + Width  bit1=sample_width * -1  base1=MSB of Input  bit0=0  base0=LSB of Input  dbl_ovrd=off  block_type=slice
      settings: block_version=11.3
  Slice3 : xbsIndex_r4/Slice  nbits=sample_width  boolean_output=off  mode=Upper Bit Location + Width  bit1=sample_width * -2  base1=MSB of Input  bit0=0  base0=LSB of Input  dbl_ovrd=off  block_type=slice
      settings: block_version=11.3
  Slice32 : xbsIndex_r4/Slice  nbits=sample_width  boolean_output=off  mode=Upper Bit Location + Width  bit1=sample_width * 0  base1=MSB of Input  bit0=0  base0=LSB of Input  dbl_ovrd=off  block_type=slice
      settings: block_version=11.3
  Slice33 : xbsIndex_r4/Slice  nbits=sample_width  boolean_output=off  mode=Upper Bit Location + Width  bit1=sample_width * -9  base1=MSB of Input  bit0=0  base0=LSB of Input  dbl_ovrd=off  block_type=slice
      settings: block_version=11.3
  Slice34 : xbsIndex_r4/Slice  nbits=sample_width  boolean_output=off  mode=Upper Bit Location + Width  bit1=sample_width * -10  base1=MSB of Input  bit0=0  base0=LSB of Input  dbl_ovrd=off  block_type=slice
      settings: block_version=11.3
  Slice35 : xbsIndex_r4/Slice  nbits=sample_width  boolean_output=off  mode=Upper Bit Location + Width  bit1=sample_width * -11  base1=MSB of Input  bit0=0  base0=LSB of Input  dbl_ovrd=off  block_type=slice
      settings: block_version=11.3
  Slice36 : xbsIndex_r4/Slice  nbits=sample_width  boolean_output=off  mode=Upper Bit Location + Width  bit1=sample_width * -12  base1=MSB of Input  bit0=0  base0=LSB of Input  dbl_ovrd=off  block_type=slice
      settings: block_version=11.3
  Slice37 : xbsIndex_r4/Slice  nbits=sample_width  boolean_output=off  mode=Upper Bit Location + Width  bit1=sample_width * -13  base1=MSB of Input  bit0=0  base0=LSB of Input  dbl_ovrd=off  block_type=slice
      settings: block_version=11.3
  Slice38 : xbsIndex_r4/Slice  nbits=sample_width  boolean_output=off  mode=Upper Bit Location + Width  bit1=sample_width * -14  base1=MSB of Input  bit0=0  base0=LSB of Input  dbl_ovrd=off  block_type=slice
      settings: block_version=11.3
  Slice39 : xbsIndex_r4/Slice  nbits=sample_width  boolean_output=off  mode=Upper Bit Location + Width  bit1=sample_width * -15  base1=MSB of Input  bit0=0  base0=LSB of Input  dbl_ovrd=off  block_type=slice
      settings: block_version=11.3
  Slice4 : xbsIndex_r4/Slice  nbits=sample_width  boolean_output=off  mode=Upper Bit Location + Width  bit1=sample_width * -3  base1=MSB of Input  bit0=0  base0=LSB of Input  dbl_ovrd=off  block_type=slice
      settings: block_version=11.3
  Slice40 : xbsIndex_r4/Slice  nbits=sample_width  boolean_output=off  mode=Upper Bit Location + Width  bit1=sample_width * -1  base1=MSB of Input  bit0=0  base0=LSB of Input  dbl_ovrd=off  block_type=slice
      settings: block_version=11.3
  Slice41 : xbsIndex_r4/Slice  nbits=sample_width  boolean_output=off  mode=Upper Bit Location + Width  bit1=sample_width * -2  base1=MSB of Input  bit0=0  base0=LSB of Input  dbl_ovrd=off  block_type=slice
      settings: block_version=11.3
  Slice42 : xbsIndex_r4/Slice  nbits=sample_width  boolean_output=off  mode=Upper Bit Location + Width  bit1=sample_width * -3  base1=MSB of Input  bit0=0  base0=LSB of Input  dbl_ovrd=off  block_type=slice
      settings: block_version=11.3
  Slice43 : xbsIndex_r4/Slice  nbits=sample_width  boolean_output=off  mode=Upper Bit Location + Width  bit1=sample_width * -4  base1=MSB of Input  bit0=0  base0=LSB of Input  dbl_ovrd=off  block_type=slice
      settings: block_version=11.3
  Slice44 : xbsIndex_r4/Slice  nbits=sample_width  boolean_output=off  mode=Upper Bit Location + Width  bit1=sample_width * -5  base1=MSB of Input  bit0=0  base0=LSB of Input  dbl_ovrd=off  block_type=slice
      settings: block_version=11.3
  Slice45 : xbsIndex_r4/Slice  nbits=sample_width  boolean_output=off  mode=Upper Bit Location + Width  bit1=sample_width * -6  base1=MSB of Input  bit0=0  base0=LSB of Input  dbl_ovrd=off  block_type=slice
      settings: block_version=11.3
  Slice46 : xbsIndex_r4/Slice  nbits=sample_width  boolean_output=off  mode=Upper Bit Location + Width  bit1=sample_width * -7  base1=MSB of Input  bit0=0  base0=LSB of Input  dbl_ovrd=off  block_type=slice
      settings: block_version=11.3
  Slice47 : xbsIndex_r4/Slice  nbits=sample_width  boolean_output=off  mode=Upper Bit Location + Width  bit1=sample_width * -8  base1=MSB of Input  bit0=0  base0=LSB of Input  dbl_ovrd=off  block_type=slice
      settings: block_version=11.3
  Slice5 : xbsIndex_r4/Slice  nbits=sample_width  boolean_output=off  mode=Upper Bit Location + Width  bit1=sample_width * -4  base1=MSB of Input  bit0=0  base0=LSB of Input  dbl_ovrd=off  block_type=slice
      settings: block_version=11.3
  Slice6 : xbsIndex_r4/Slice  nbits=sample_width  boolean_output=off  mode=Upper Bit Location + Width  bit1=sample_width * -5  base1=MSB of Input  bit0=0  base0=LSB of Input  dbl_ovrd=off  block_type=slice
      settings: block_version=11.3
  Slice7 : xbsIndex_r4/Slice  nbits=sample_width  boolean_output=off  mode=Upper Bit Location + Width  bit1=sample_width * -6  base1=MSB of Input  bit0=0  base0=LSB of Input  dbl_ovrd=off  block_type=slice
      settings: block_version=11.3
  Slice8 : xbsIndex_r4/Slice  nbits=sample_width  boolean_output=off  mode=Upper Bit Location + Width  bit1=sample_width * -7  base1=MSB of Input  bit0=0  base0=LSB of Input  dbl_ovrd=off  block_type=slice
      settings: block_version=11.3
  Slice9 : xbsIndex_r4/Slice  nbits=sample_width  boolean_output=off  mode=Upper Bit Location + Width  bit1=sample_width * -8  base1=MSB of Input  bit0=0  base0=LSB of Input  dbl_ovrd=off  block_type=slice
      settings: block_version=11.3
  wires:
  bs1/1 -> Slice16/1, Slice15/1, Slice14/1, Slice13/1, Slice12/1, Slice11/1, Slice10/1, Slice9/1, Slice8/1, Slice7/1, Slice6/1, Slice5/1, Slice4/1, Slice3/1, Slice2/1, Slice1/1
  Multiport Switch1/1 -> Scope/3
  Multiport Switch/1 -> Scope/2
  Gateway Out8/1 -> Scope/1
  sync/1 -> Gateway Out8/1
  Gateway Out25/1 -> Multiport Switch1/17
  Gateway Out24/1 -> Multiport Switch1/16
  Gateway Out23/1 -> Multiport Switch1/15
  Gateway Out22/1 -> Multiport Switch1/14
  Gateway Out21/1 -> Multiport Switch1/13
  Gateway Out20/1 -> Multiport Switch1/12
  Gateway Out19/1 -> Multiport Switch1/11
  Gateway Out32/1 -> Multiport Switch1/10
  Gateway Out31/1 -> Multiport Switch1/9
  Gateway Out30/1 -> Multiport Switch1/8
  Gateway Out29/1 -> Multiport Switch1/7
  Gateway Out28/1 -> Multiport Switch1/6
  Gateway Out27/1 -> Multiport Switch1/5
  Gateway Out26/1 -> Multiport Switch1/4
  Gateway Out18/1 -> Multiport Switch1/3
  Gateway Out17/1 -> Multiport Switch1/2
  Gateway Out16/1 -> Multiport Switch/17
  Gateway Out15/1 -> Multiport Switch/16
  Gateway Out14/1 -> Multiport Switch/15
  Gateway Out13/1 -> Multiport Switch/14
  Gateway Out12/1 -> Multiport Switch/13
  Gateway Out11/1 -> Multiport Switch/12
  Gateway Out10/1 -> Multiport Switch/11
  Gateway Out9/1 -> Multiport Switch/10
  Gateway Out7/1 -> Multiport Switch/9
  Gateway Out6/1 -> Multiport Switch/8
  Gateway Out5/1 -> Multiport Switch/7
  Gateway Out4/1 -> Multiport Switch/6
  Gateway Out3/1 -> Multiport Switch/5
  Gateway Out2/1 -> Multiport Switch/4
  Gateway Out1/1 -> Multiport Switch/3
  Gateway Out/1 -> Multiport Switch/2
  Slice9/1 -> Gateway Out32/1
  Slice10/1 -> Gateway Out19/1
  Slice11/1 -> Gateway Out20/1
  Slice12/1 -> Gateway Out21/1
  Slice13/1 -> Gateway Out22/1
  Slice14/1 -> Gateway Out23/1
  Slice15/1 -> Gateway Out24/1
  Slice16/1 -> Gateway Out25/1
  Slice1/1 -> Gateway Out17/1
  Slice2/1 -> Gateway Out18/1
  Slice3/1 -> Gateway Out26/1
  Slice4/1 -> Gateway Out27/1
  Slice5/1 -> Gateway Out28/1
  Slice6/1 -> Gateway Out29/1
  Slice7/1 -> Gateway Out30/1
  Slice8/1 -> Gateway Out31/1
  Slice47/1 -> Gateway Out9/1
  Slice33/1 -> Gateway Out10/1
  Slice34/1 -> Gateway Out11/1
  Slice35/1 -> Gateway Out12/1
  Slice36/1 -> Gateway Out13/1
  Slice37/1 -> Gateway Out14/1
  Slice38/1 -> Gateway Out15/1
  Slice39/1 -> Gateway Out16/1
  bs0/1 -> Slice32/1, Slice40/1, Slice41/1, Slice42/1, Slice43/1, Slice44/1, Slice45/1, Slice46/1, Slice47/1, Slice33/1, Slice34/1, Slice35/1, Slice36/1, Slice37/1, Slice39/1, Slice38/1
  Slice32/1 -> Gateway Out/1
  Slice40/1 -> Gateway Out1/1
  Slice41/1 -> Gateway Out2/1
  Slice42/1 -> Gateway Out3/1
  Slice43/1 -> Gateway Out4/1
  Slice44/1 -> Gateway Out5/1
  Slice45/1 -> Gateway Out6/1
  Slice46/1 -> Gateway Out7/1
  Counter Free-Running/1 -> Multiport Switch1/1, Multiport Switch/1

== system dbe_xaui_corr_32X/noise ==
  note: These are the "seed" and "arm" control registers for the
      | noise generator, which lives in the input_mux block.
  Constant10 : Constant  Value=0
  Constant11 : Constant  Value=0
  arm : xps_library/software register  Tag=xps:sw_reg  SystemSampleTime=-1  io_dir=From Processor  arith_type=Unsigned  bitwidth=32  bin_pt=0  sample_period=1  gw_name=dbe_xaui_corr_32X_noise_arm_user_data_out
      link override dbe_adc_single_noise_arm_user_data_out: arith_type=Unsigned  n_bits=32  bin_pt=0  period=1
      link override dbe_adc_single_shiftctrl_reg_user_data_out: arith_type=Unsigned  n_bits=32  bin_pt=0  period=1
      link override dbe_xaui_corr_32X_noise_arm_user_data_out: arith_type=Unsigned  n_bits=32  bin_pt=0  period=1
      link override vlbipfb2_m3_ibob_shiftctrl_reg_user_data_out: arith_type=Unsigned  n_bits=32  bin_pt=0  period=1
      link override vlbipfb2_m3_roach_shiftctrl_reg_user_data_out: arith_type=Unsigned  n_bits=32  bin_pt=0  period=1
  seed : xps_library/software register  Tag=xps:sw_reg  SystemSampleTime=-1  io_dir=From Processor  arith_type=Unsigned  bitwidth=32  bin_pt=0  sample_period=1  gw_name=dbe_xaui_corr_32X_noise_seed_user_data_out
      link override dbe_adc_single_noise_seed_user_data_out: arith_type=Unsigned  n_bits=32  bin_pt=0  period=1
      link override dbe_adc_single_shiftctrl_reg_user_data_out: arith_type=Unsigned  n_bits=32  bin_pt=0  period=1
      link override dbe_xaui_corr_32X_noise_seed_user_data_out: arith_type=Unsigned  n_bits=32  bin_pt=0  period=1
      link override vlbipfb2_m3_ibob_shiftctrl_reg_user_data_out: arith_type=Unsigned  n_bits=32  bin_pt=0  period=1
      link override vlbipfb2_m3_roach_shiftctrl_reg_user_data_out: arith_type=Unsigned  n_bits=32  bin_pt=0  period=1
  tag scope: wgn_arm=global, wgn_seed=global
  wires:
  seed/1 -> [wgn_seed]
  arm/1 -> [wgn_arm]
  Constant10/1 -> arm/1
  Constant11/1 -> seed/1
